simulink model "uniqueWordBatch"  (R2018b)
settings: Solver=FixedStepDiscrete  StartTime=0.0  StopTime=inf  RelTol=1e-3
values from neighbouring files (symbols this model uses):
  EbNo = 8:15    [symulujUWvsDiff.m]
libraries: commutil2 x2, commdigbbndpm3 x2, commfilt2 x2, commchan3 x1, simulink x1, dspstat3 x1, commrandsrc3 x1, commsink2 x1, commrflib2 x1, dspsigops x1
settings Model: Creator=sikor  LastModifiedBy=sikor
settings SolverCC: AlgebraicLoopSolver=LineSearch
settings OptimizationCC: LifeSpan=inf
settings DebuggingCC: SFUnexpectedBacktrackingDiag=warning  SFNoUnconditionalDefaultTransitionDiag=warning
settings SFSimCC: SimUseLocalCustomCode=off
settings RTWCC: RTWUseLocalCustomCode=off
settings CodeAppCC: StateflowObjectComments=on
settings GRTTargetCC: TargetLangStandard=C89/C90 (ANSI)  GeneratePreprocessorConditionals=Disable all
settings ConfigComp: CovMetricSettings=dw  CovHtmlReporting=on  CovSaveCumulativeToWorkspaceVar=on  CovSaveSingleToWorkspaceVar=on  CovExternalEMLEnable=off

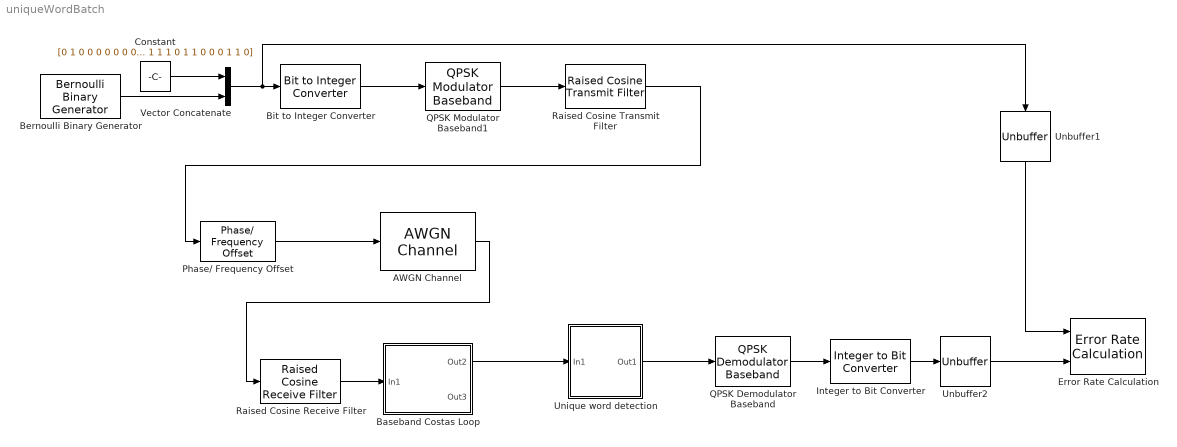
== system uniqueWordBatch ==
  AWGN Channel : commchan3/AWGN Channel  InputProcessing=Columns as channels (frame based)  seed=67  noiseMode="Signal to noise ratio  (Eb/No)"  EbNodB=EbNo  EsNodB=10  SNRdB=10  bitsPerSym=2  Ps=1  Tsym=1  variance=1
      settings: SourceProductName=Communications Toolbox
  Baseband Costas Loop : Subsystem  mask{loopBw=2.0*pi/200.0, sampleTime=1}
      mask prompts: loopBw "Select loop bandwidth"; sampleTime "Sample time"
      mask init:
      | damp=0.707;
      | %set_param('costasLoop','AlgebraicLoopSolver','TrustRegion')
      | alpha = (4.0 * damp * loopBw) / (1.0 + 2.0 * damp * loopBw + loopBw * loopBw); 
      | beta = (4.0 * loopBw * loopBw) / (1.0 + 2.0 * damp * loopBw + loopBw * loopBw); 
      | set_param(sprintf('%s/Baseband Costas Loop/Alfa',gcs),'Gain',sprintf('%f',alpha))
      | set_param(sprintf('%s/Baseband Costas Loop/Beta',gcs),'Gain',sprintf('%f',beta))
      | %set_param(sprintf('%s/Baseband Costas Loop/Mean1',gcs),'Ts',sprintf('%f',sampleTime))
      mask Display: disp('Costas\nLoop');
  Bernoulli Binary Generator : commrandsrc3/Bernoulli Binary Generator  ProbabilityOfZero=0.5  SeedSource=Auto  Seed=0  SampleTime=240  SamplesPerFrame=480  OutputDataType=uint8  SimulateUsing=Interpreted execution
      settings: SourceProductName=Communications Toolbox
  Bit to Integer Converter : commutil2/Bit to Integer Converter  nbits=2  bitOrder=MSB first  signedOutputValues=Unsigned  outDtype=int16  outDtypeSigned=Inherit via internal rule
      settings: SourceProductName=Communications Toolbox
  Constant : Constant  Value=[0 1 0 0 0 0 0 0 0 1 1 1 0 0 0 0 0 1 0 0 1 1 1 0 1 1 0 0 0 1 1 0]  OutDataTypeStr=uint8  SampleTime=240
  Error Rate Calculation : commsink2/Error Rate Calculation  N=532  st_delay=1000  cp_mode=Entire frame  subframe=[]  PMode=Workspace  WsName=BER  RsMode2=off  stop=on  numErr=maxNumErrs  maxBits=maxNumBits
      settings: SourceProductName=Communications Toolbox
  Integer to Bit Converter : commutil2/Integer to Bit Converter  nbits=2  signedInputValues=Unsigned  bitOrder=MSB first  outDtype=Inherit via internal rule
      settings: SourceProductName=Communications Toolbox
  Phase/ Frequency Offset : commrflib2/Phase// Frequency Offset  phaseOffset=40  freqPort=off  freqOffset=.0045
      settings: SourceProductName=Communications Toolbox
  QPSK Demodulator Baseband : commdigbbndpm3/QPSK Demodulator Baseband  OutType=Integer  DecType=Hard decision  VarSource=Dialog  Variance=1  Dec=Gray  Ph=pi/4  outDtype1=Inherit via internal rule  outDtype2=int16  derotateFactorWordLen=16  derotateFactorDataTypeStr=Inherit: Same word length as input  derotateFactorLastDataTypeStr=Inherit: Same word length as input
      settings: SourceProductName=Communications Toolbox
  QPSK Modulator Baseband1 : commdigbbndpm3/QPSK Modulator Baseband  InType=Integer  Enc=Gray  Ph=pi/4  outDtype=double  outWordLen=16  outUDDataType=sfix(16)  outFracLenMode=Best precision  outFracLen=15  outDataTypeStr=double  outLastDataTypeStr=double
      settings: SourceProductName=Communications Toolbox
  Raised Cosine Receive Filter : commfilt2/Raised Cosine Receive Filter  filtType=Square root  R=0.2  filtSpan=10  N=4  downFactor=4  downOffset=0  filterGain=1  InputProcessing=Columns as channels (frame based)  RateOptions=Allow multirate processing  framing=Mute  checkCoeff=off  variableName=rcRxFilt  currentFiltSpan=10  D=5  inputOffset=0  sampMode=Mute  saveAsFlag=0  rateMode=Downsampling  checkGain=Normalized  launchFVT=on  roundingMode=Floor  overflowMode=off  coeffDataTypeStr=Inherit: Same word length as input  coeffMin=[]  coeffMax=[]  coeffLastDataTypeStr=Inherit: Same word length as input  accumDataTypeStr=Inherit: Same as product output  accumLastDataTypeStr=Inherit: Same as product output  outputDataTypeStr=Inherit: Same as accumulator  outputMin=[]  outputMax=[]  outputLastDataTypeStr=Inherit: Same as accumulator
      settings: SourceProductName=Communications Toolbox
  Raised Cosine Transmit Filter : commfilt2/Raised Cosine Transmit Filter  filtType=Square root  R=0.2  filtSpan=10  N=4  filterGain=1  InputProcessing=Columns as channels (frame based)  RateOptions=Allow multirate processing  framing=Mute  checkCoeff=off  variableName=rcTxFilt  checkGain=Normalized  sampMode=Mute  saveAsFlag=0  currentFiltSpan=10  D=5  launchFVT=on  roundingMode=Floor  overflowMode=off  coeffDataTypeStr=Inherit: Same word length as input  coeffMin=[]  coeffMax=[]  coeffLastDataTypeStr=Inherit: Same word length as input  outputDataTypeStr=Inherit: Same as accumulator  outputMin=[]  outputMax=[]  outputLastDataTypeStr=Inherit: Same as accumulator
      settings: SourceProductName=Communications Toolbox
  Unbuffer1 : Unbuffer
  Unbuffer2 : Unbuffer
  Unique word detection : Subsystem
      mask Display: disp('Detect phase\nshift')
  Vector Concatenate : Concatenate
  wires:
  Constant/1 -> Vector Concatenate/1
  Bernoulli Binary Generator/1 -> Vector Concatenate/2
  Vector Concatenate/1 -> Unbuffer1/1, Bit to Integer Converter/1
  Raised Cosine Transmit Filter/1 -> Phase/ Frequency Offset/1
  QPSK Modulator Baseband1/1 -> Raised Cosine Transmit Filter/1
  Bit to Integer Converter/1 -> QPSK Modulator Baseband1/1
  Raised Cosine Receive Filter/1 -> Baseband Costas Loop/1(In1)
  Baseband Costas Loop/1(Out2) -> Unique word detection/1(In1)
  Unique word detection/1(Out1) -> QPSK Demodulator Baseband/1
  QPSK Demodulator Baseband/1 -> Integer to Bit Converter/1
  Unbuffer1/1 -> Error Rate Calculation/1
  Integer to Bit Converter/1 -> Unbuffer2/1
  Unbuffer2/1 -> Error Rate Calculation/2
  Phase/ Frequency Offset/1 -> AWGN Channel/1
  AWGN Channel/1 -> Raised Cosine Receive Filter/1

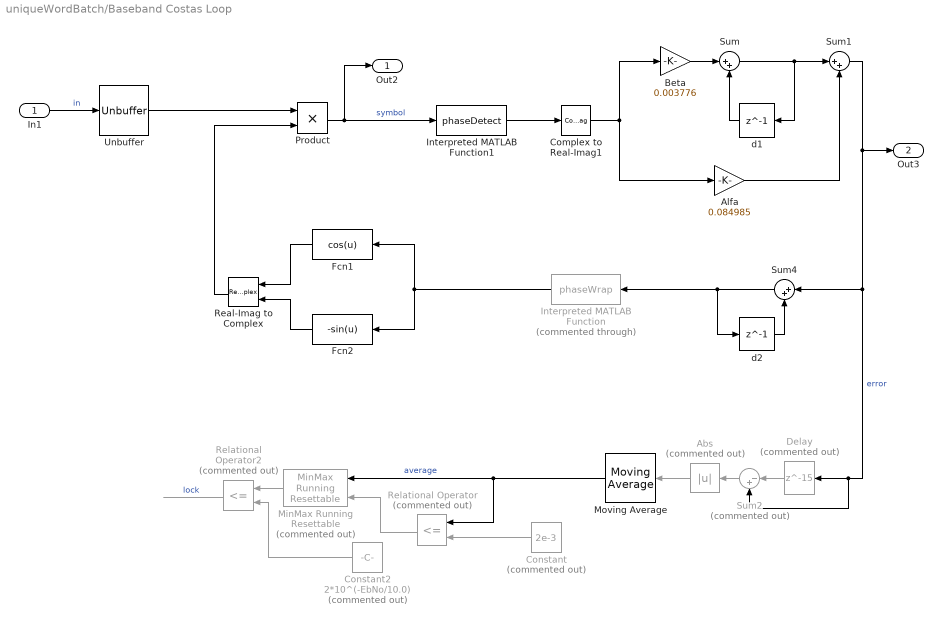
== system uniqueWordBatch/Baseband Costas Loop ==
  In1 : Inport
  Abs : Abs  Commented=on
  Alfa : Gain  Gain=0.084985
  Beta : Gain  Gain=0.003776
  Complex to Real-Imag1 : ComplexToRealImag  Output=Real
  Constant : Constant  Commented=on  Value=2e-3
  Constant2 : Constant  Commented=on  Value=2*10^(-EbNo/10.0)
  Delay : Delay  Commented=on  DelayLength=15  InitialCondition=0
  Fcn1 : Fcn  Expr=cos(u)
  Fcn2 : Fcn  Expr=-sin(u)
  Interpreted MATLAB Function : MATLABFcn  Commented=through  MATLABFcn=phaseWrap
  Interpreted MATLAB Function1 : MATLABFcn  MATLABFcn=phaseDetect
  MinMax Running Resettable : simulink/Math Operations/MinMax Running Resettable  Commented=on  Function=max  vinit=0.0
  Moving Average : dspstat3/Moving Average  Method=Exponential weighting  ForgettingFactorPort=off  SpecifyWindowLength=on  WindowLength=64  ForgettingFactor=0.9  SimulateUsing=Code generation
  Product : Product  OutDataTypeStr=double  RndMeth=Round
  Real-Imag to Complex : RealImagToComplex
  Relational Operator : RelationalOperator  Commented=on  Operator=<=  OutDataTypeStr=boolean  RndMeth=Nearest
  Relational Operator2 : RelationalOperator  Commented=on  Operator=<=  OutDataTypeStr=boolean  RndMeth=Nearest
  Sum : Sum  Inputs=|++  OutDataTypeStr=double  RndMeth=Round
  Sum1 : Sum  Inputs=|++  OutDataTypeStr=double  RndMeth=Nearest
  Sum2 : Sum  Commented=on  Inputs=|-+
  Sum4 : Sum  Inputs=|++
  Unbuffer : Unbuffer
  d1 : Delay  DelayLength=1  InitialCondition=0
  d2 : Delay  DelayLength=1  InitialCondition=0
  Out2 : Outport
  Out3 : Outport  Port=2
  wires:
  In1/1 -> Unbuffer/1  "in"
  d1/1 -> Sum/2
  Sum/1 -> d1/1, Sum1/1
  Alfa/1 -> Sum1/2
  Beta/1 -> Sum/1
  Product/1 -> Out2/1, Interpreted MATLAB Function1/1  "symbol"
  Real-Imag to Complex/1 -> Product/2
  Unbuffer/1 -> Product/1
  Sum4/1 -> d2/1, Interpreted MATLAB Function/1
  d2/1 -> Sum4/2
  Interpreted MATLAB Function/1 -> Fcn1/1, Fcn2/1
  Fcn1/1 -> Real-Imag to Complex/1
  Fcn2/1 -> Real-Imag to Complex/2
  Sum1/1 -> Sum2/2, Delay/1, Sum4/1, Out3/1  "error"
  Interpreted MATLAB Function1/1 -> Complex to Real-Imag1/1
  Complex to Real-Imag1/1 -> Alfa/1, Beta/1
  Constant2/1 -> Relational Operator2/2
  Delay/1 -> Sum2/1
  Constant/1 -> Relational Operator/2
  Sum2/1 -> Abs/1
  Moving Average/1 -> MinMax Running Resettable/1, Relational Operator/1  "average"
  Relational Operator/1 -> MinMax Running Resettable/2
  MinMax Running Resettable/1 -> Relational Operator2/1
  Abs/1 -> Moving Average/1
  Relational Operator2/1 -> ?  "lock"

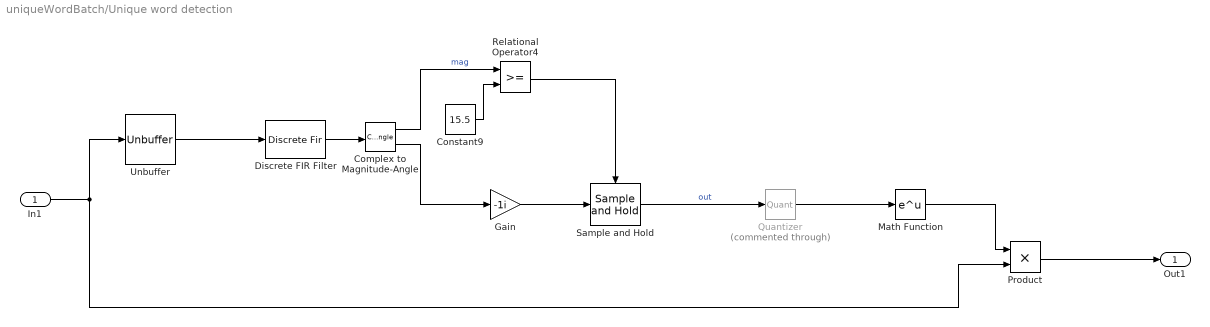
== system uniqueWordBatch/Unique word detection ==
  In1 : Inport
  Complex to Magnitude-Angle : ComplexToMagnitudeAngle
  Constant9 : Constant  Value=15.5
  Discrete FIR Filter : DiscreteFir  Coefficients=[0.707+0.707i;-0.707-0.707i;0.707-0.707i;-0.707+0.707i;0.707+0.707i;-0.707+0.707i;0.707-0.707i;-0.707-0.707i;0.707-0.707i;0.707-0.707i;-0.707+0.707i;-0.707-0.707i;0.707-0.707i;0.707-0.707i;0.707-0.707i;-0.707-0.707i].'
  Gain : Gain  Gain=-1i
  Math Function : Math  SaturateOnIntegerOverflow=on
  Product : Product
  Quantizer : Quantizer  Commented=through  QuantizationInterval=0.5*pi
  Relational Operator4 : RelationalOperator  OutDataTypeStr=boolean  RndMeth=Nearest
  Sample and Hold : dspsigops/Sample and Hold  trig=Rising edge  initCond=0  latchinput=off
  Unbuffer : Unbuffer
  Out1 : Outport
  wires:
  Relational Operator4/1 -> Sample and Hold/Trigger
  Constant9/1 -> Relational Operator4/2
  In1/1 -> Unbuffer/1, Product/2
  Discrete FIR Filter/1 -> Complex to Magnitude-Angle/1
  Complex to Magnitude-Angle/1 -> Relational Operator4/1  "mag"
  Complex to Magnitude-Angle/2 -> Gain/1
  Gain/1 -> Sample and Hold/1
  Math Function/1 -> Product/1
  Product/1 -> Out1/1
  Unbuffer/1 -> Discrete FIR Filter/1
  Quantizer/1 -> Math Function/1
  Sample and Hold/1 -> Quantizer/1  "out"
